simulink model "encoderRPM"  (R2019b)
settings: Solver=FixedStepAuto  StartTime=0.0  StopTime=inf  RelTol=1e-3
libraries: arduinolib x3, eeQuadratureDecoder x1
settings Model: SILPILModeSetting=veronly  ExtModeTrigDuration=2  Creator=covasanvictor  LastModifiedBy=covasanvictor
settings OptimizationCC: EnhancedBackFolding=on  PassReuseOutputArgsAs=Individual arguments  ZeroExternalMemoryAtStartup=off  ZeroInternalMemoryAtStartup=off  MaxStackSize=64  OptimizeBlockOrder=speed  DifferentSizesBufferReuse=on  OptimizationCustomize=off  EfficientTunableParamExpr=on
settings DebuggingCC: ParameterTunabilityLossMsg=error
settings HardwareCC: ProdBitPerInt=16  ProdBitPerPointer=16  ProdBitPerSizeT=16  ProdBitPerPtrDiffT=16  ProdLargestAtomicFloat=None  ProdWordSize=8  ProdHWDeviceType=Atmel->AVR  UseEmbeddedCoderFeatures=off  UseSimulinkCoderFeatures=off
settings SFSimCC: MATLABDynamicMemAlloc=off
settings RTWCC: SystemTargetFile=ert.tlc  HardwareBoard=Arduino Uno  TLCOptions=-aInlineSetEventsForThisBaseRateFcn=TLC_FALSE -aSuppressMultiTaskScheduler=TLC_FALSE -aRateBasedStepFcn=1  TemplateMakefile=ert_default_tmf  GenerateReport=on  Toolchain=Arduino AVR  IncludeHyperlinkInReport=on  LaunchReport=on  GenerateTraceInfo=on  GenerateTraceReport=on  GenerateTraceReportSl=on  GenerateTraceReportSf=on  GenerateTraceReportEml=on
settings CodeAppCC: ForceParamTrailComments=on  IgnoreCustomStorageClasses=off  OperatorAnnotations=on  SimulinkDataObjDesc=on  SFDataObjDesc=on  InsertBlockDesc=on
settings ERTTargetCC: SupportContinuousTime=on  SupportNonInlinedSFcns=on  SupportVariableSizeSignals=on  ExtModeStaticAllocSize=250

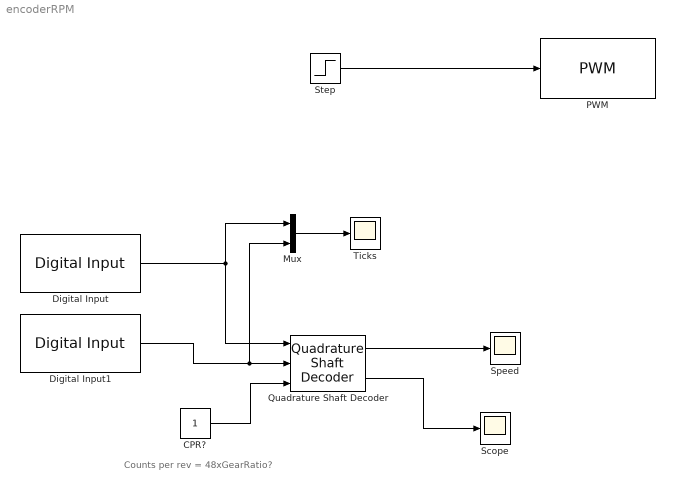
== system encoderRPM ==
  note: Counts per rev = 48xGearRatio?
  CPR? : Constant
  Digital Input : arduinolib/Digital Input  pinNumber=2  SampleTime=-1  blockPlatform=arduino
      settings: SourceProductName=Simulink Support Package for Arduino Hardware
  Digital Input1 : arduinolib/Digital Input  pinNumber=3  SampleTime=-1  blockPlatform=arduino
      settings: SourceProductName=Simulink Support Package for Arduino Hardware
  Mux : Mux  Inputs=2
  PWM : arduinolib/PWM  pinNumber=6  EnableInputFrequency=off  InitialFrequency=2000  InitialDutyCycle=0  NotificationType=None  blockPlatform=arduino
  Quadrature Shaft Decoder : eeQuadratureDecoder/Quadrature Shaft Decoder  NPulse=48  Ts=-1
      settings: SourceProductName=Simscape Electrical  SourceProductBaseCode=PS
  Scope : Scope
  Speed : Scope
  Step : Step  After=255  SampleTime=0
  Ticks : Scope
  wires:
  Step/1 -> PWM/1
  Digital Input/1 -> Mux/1, Quadrature Shaft Decoder/1
  Digital Input1/1 -> Mux/2, Quadrature Shaft Decoder/2
  CPR?/1 -> Quadrature Shaft Decoder/3
  Quadrature Shaft Decoder/1 -> Speed/1
  Quadrature Shaft Decoder/2 -> Scope/1
  Mux/1 -> Ticks/1
